simulink model "battery_simulink_model"  (R2021b)
settings: Solver=VariableStepAuto  StartTime=0.0  StopTime=14400  RelTol=1e-3
undefined symbols (not defined in the file or in its folder): Ion, Lithium
libraries: spsBatteryLib x10, spsIdealSwitchLib x4, spsCurrentMeasurementLib x3, spsParallelRLCBranchLib x2, spsControlledCurrentSourceLib x1, spspowerguiLib x1
settings Model: Creator=11  LastModifiedBy=11

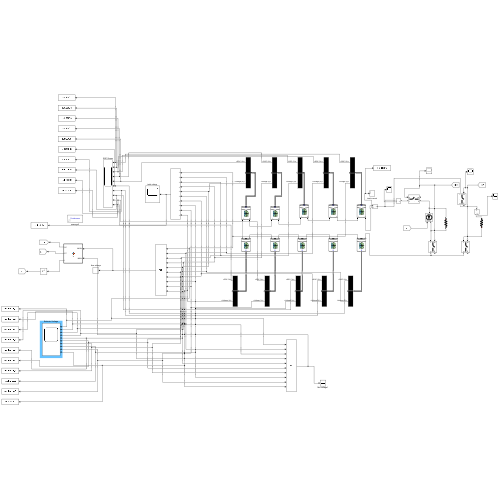
[thumbnail: Simulink's stored preview of the top-level diagram]
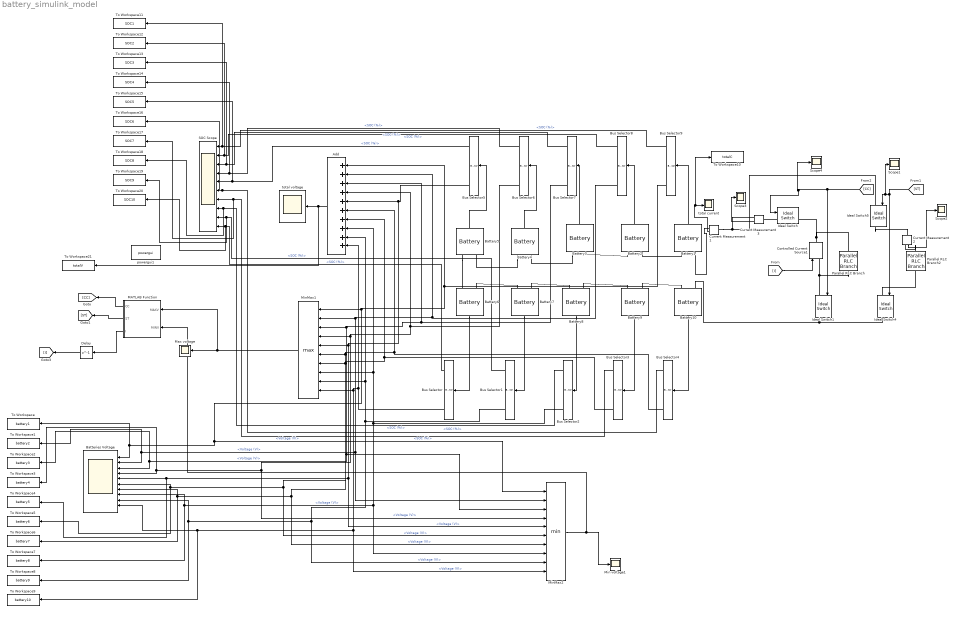
== system battery_simulink_model ==
  Add : Sum  Inputs=++++++++++
  Batteries Voltage : Scope  NumInputPorts=10
  Battery1 : spsBatteryLib/Battery  BatType=Lithium-Ion  ShowTempParam=off  ThermalPreset=no  ShowAgeParam=off  NomV=3.2  NomQ=226.1  SOC=5  Batt_Tr=30  PresetModel=off  MaxQ=226.1  MinV=2.5  FullV=3.65  Dis_rate=114  R=0.0002289  Normal_OP=203.49  expZone=[3.45,10]  current=[114]  Units=Time  Tci=20  NomT=20  T2=-30  MaxQ2=4.8  FullV2=7.1  Normal_OP2=5.655  expZone2="[6.58           1]"  Rca=0.6  ti=2000  Dp=0  Neq0=0  Tsim=1e6  Ta1=25  Qeol=5.4*0.9  Reol=0.013333*1.2  Char_age=[2.3478, 3]  Dis_age=[2.3478, 10]  N1=1500  N2=10500  N3=1000  N4=1400  Ta2=45  N5=950
  Battery10 : spsBatteryLib/Battery  BatType=Lithium-Ion  ShowTempParam=off  ThermalPreset=no  ShowAgeParam=off  NomV=3.2  NomQ=233.3  SOC=11  Batt_Tr=30  PresetModel=off  MaxQ=233.3  MinV=2.5  FullV=3.65  Dis_rate=114  R=0.0002189  Normal_OP=209.97  expZone=[3.45,10]  current=[114]  Units=Time  Tci=20  NomT=20  T2=-30  MaxQ2=4.8  FullV2=7.1  Normal_OP2=5.655  expZone2="[6.58           1]"  Rca=0.6  ti=2000  Dp=0  Neq0=0  Tsim=1e6  Ta1=25  Qeol=5.4*0.9  Reol=0.013333*1.2  Char_age=[2.3478, 3]  Dis_age=[2.3478, 10]  N1=1500  N2=10500  N3=1000  N4=1400  Ta2=45  N5=950
  Battery2 : spsBatteryLib/Battery  BatType=Lithium-Ion  ShowTempParam=off  ThermalPreset=no  ShowAgeParam=off  NomV=3.2  NomQ=238.1  SOC=10  Batt_Tr=30  PresetModel=off  MaxQ=238.1  MinV=2.5  FullV=3.65  Dis_rate=114  R=0.0002198  Normal_OP=214.29  expZone=[3.45,10]  current=[114]  Units=Time  Tci=20  NomT=20  T2=-30  MaxQ2=4.8  FullV2=7.1  Normal_OP2=5.655  expZone2="[6.58           1]"  Rca=0.6  ti=2000  Dp=0  Neq0=0  Tsim=1e6  Ta1=25  Qeol=5.4*0.9  Reol=0.013333*1.2  Char_age=[2.3478, 3]  Dis_age=[2.3478, 10]  N1=1500  N2=10500  N3=1000  N4=1400  Ta2=45  N5=950
  Battery3 : spsBatteryLib/Battery  BatType=Lithium-Ion  ShowTempParam=off  ThermalPreset=no  ShowAgeParam=off  NomV=3.2  NomQ=224.3  SOC=14  Batt_Tr=30  PresetModel=off  MaxQ=224.3  MinV=2.5  FullV=3.65  Dis_rate=114  R=0.0002171  Normal_OP=201.87  expZone=[3.45,10]  current=[114]  Units=Time  Tci=20  NomT=20  T2=-30  MaxQ2=4.8  FullV2=7.1  Normal_OP2=5.655  expZone2="[6.58           1]"  Rca=0.6  ti=2000  Dp=0  Neq0=0  Tsim=1e6  Ta1=25  Qeol=5.4*0.9  Reol=0.013333*1.2  Char_age=[2.3478, 3]  Dis_age=[2.3478, 10]  N1=1500  N2=10500  N3=1000  N4=1400  Ta2=45  N5=950
  Battery4 : spsBatteryLib/Battery  BatType=Lithium-Ion  ShowTempParam=off  ThermalPreset=no  ShowAgeParam=off  NomV=3.2  NomQ=219.1  SOC=13  Batt_Tr=30  PresetModel=off  MaxQ=219.1  MinV=2.5  FullV=3.65  Dis_rate=114  R=0.0002176  Normal_OP=197.19  expZone=[3.45,10]  current=[114]  Units=Time  Tci=20  NomT=20  T2=-30  MaxQ2=4.8  FullV2=7.1  Normal_OP2=5.655  expZone2="[6.58           1]"  Rca=0.6  ti=2000  Dp=0  Neq0=0  Tsim=1e6  Ta1=25  Qeol=5.4*0.9  Reol=0.013333*1.2  Char_age=[2.3478, 3]  Dis_age=[2.3478, 10]  N1=1500  N2=10500  N3=1000  N4=1400  Ta2=45  N5=950
  Battery5 : spsBatteryLib/Battery  BatType=Lithium-Ion  ShowTempParam=off  ThermalPreset=no  ShowAgeParam=off  NomV=3.2  NomQ=222.1  SOC=9  Batt_Tr=30  PresetModel=off  MaxQ=222.1  MinV=2.5  FullV=3.65  Dis_rate=114  R=0.0002111  Normal_OP=199.89  expZone=[3.45,10]  current=[114]  Units=Time  Tci=20  NomT=20  T2=-30  MaxQ2=4.8  FullV2=7.1  Normal_OP2=5.655  expZone2="[6.58           1]"  Rca=0.6  ti=2000  Dp=0  Neq0=0  Tsim=1e6  Ta1=25  Qeol=5.4*0.9  Reol=0.013333*1.2  Char_age=[2.3478, 3]  Dis_age=[2.3478, 10]  N1=1500  N2=10500  N3=1000  N4=1400  Ta2=45  N5=950
  Battery6 : spsBatteryLib/Battery  BatType=Lithium-Ion  ShowTempParam=off  ThermalPreset=no  ShowAgeParam=off  NomV=3.2  NomQ=219.6  SOC=14  Batt_Tr=30  PresetModel=off  MaxQ=219.6  MinV=2.5  FullV=3.65  Dis_rate=114  R=0.00023  Normal_OP=197.64  expZone=[3.45,10]  current=[114]  Units=Time  Tci=20  NomT=20  T2=-30  MaxQ2=4.8  FullV2=7.1  Normal_OP2=5.655  expZone2="[6.58           1]"  Rca=0.6  ti=2000  Dp=0  Neq0=0  Tsim=1e6  Ta1=25  Qeol=5.4*0.9  Reol=0.013333*1.2  Char_age=[2.3478, 3]  Dis_age=[2.3478, 10]  N1=1500  N2=10500  N3=1000  N4=1400  Ta2=45  N5=950
  Battery7 : spsBatteryLib/Battery  BatType=Lithium-Ion  ShowTempParam=off  ThermalPreset=no  ShowAgeParam=off  NomV=3.2  NomQ=229.7  SOC=6  Batt_Tr=30  PresetModel=off  MaxQ=229.7  MinV=2.5  FullV=3.65  Dis_rate=114  R=0.0002142  Normal_OP=206.73  expZone=[3.45,10]  current=[114]  Units=Time  Tci=20  NomT=20  T2=-30  MaxQ2=4.8  FullV2=7.1  Normal_OP2=5.655  expZone2="[6.58           1]"  Rca=0.6  ti=2000  Dp=0  Neq0=0  Tsim=1e6  Ta1=25  Qeol=5.4*0.9  Reol=0.013333*1.2  Char_age=[2.3478, 3]  Dis_age=[2.3478, 10]  N1=1500  N2=10500  N3=1000  N4=1400  Ta2=45  N5=950
  Battery8 : spsBatteryLib/Battery  BatType=Lithium-Ion  ShowTempParam=off  ThermalPreset=no  ShowAgeParam=off  NomV=3.2  NomQ=224.7  SOC=13  Batt_Tr=30  PresetModel=off  MaxQ=224.7  MinV=2.5  FullV=3.65  Dis_rate=114  R=0.0002093  Normal_OP=202.23  expZone=[3.45,10]  current=[114]  Units=Time  Tci=20  NomT=20  T2=-30  MaxQ2=4.8  FullV2=7.1  Normal_OP2=5.655  expZone2="[6.58           1]"  Rca=0.6  ti=2000  Dp=0  Neq0=0  Tsim=1e6  Ta1=25  Qeol=5.4*0.9  Reol=0.013333*1.2  Char_age=[2.3478, 3]  Dis_age=[2.3478, 10]  N1=1500  N2=10500  N3=1000  N4=1400  Ta2=45  N5=950
  Battery9 : spsBatteryLib/Battery  BatType=Lithium-Ion  ShowTempParam=off  ThermalPreset=no  ShowAgeParam=off  NomV=3.2  NomQ=217.6  SOC=7  Batt_Tr=30  PresetModel=off  MaxQ=217.6  MinV=2.5  FullV=3.65  Dis_rate=114  R=0.0002233  Normal_OP=195.84  expZone=[3.45,10]  current=[114]  Units=Time  Tci=20  NomT=20  T2=-30  MaxQ2=4.8  FullV2=7.1  Normal_OP2=5.655  expZone2="[6.58           1]"  Rca=0.6  ti=2000  Dp=0  Neq0=0  Tsim=1e6  Ta1=25  Qeol=5.4*0.9  Reol=0.013333*1.2  Char_age=[2.3478, 3]  Dis_age=[2.3478, 10]  N1=1500  N2=10500  N3=1000  N4=1400  Ta2=45  N5=950
  Bus Selector{,1..9} (10 alike) : BusSelector  OutputSignals=SOC (%),Current (A),Voltage (V)
  Controlled Current Source1 : spsControlledCurrentSourceLib/Controlled Current Source  Initialize=on  Source_Type=DC  Amplitude=0  Phase=0  Frequency=0  Measurements=None
  Current Measurement1 : spsCurrentMeasurementLib/Current Measurement  PhasorSimulation=off  OutputType=Complex  PSBequivalent=0
  Current Measurement2 : spsCurrentMeasurementLib/Current Measurement  PhasorSimulation=off  OutputType=Complex  PSBequivalent=0
  Current Measurement3 : spsCurrentMeasurementLib/Current Measurement  PhasorSimulation=off  OutputType=Complex  PSBequivalent=0
  Delay : Delay  DelayLength=1  InitialCondition=0
  Ideal Switch{,1,4..5} (4 alike) : spsIdealSwitchLib/Ideal Switch  Ron=0  Lon=0  IC=0  Rs=0  Cs=0  Measurements=on
  MATLAB Function : MATLAB Function  TreatAsAtomicUnit=on  SystemSampleTime=1
  Max voltage : Scope
  Min voltage1 : Scope
  MinMax1 : MinMax  Function=max  Inputs=10
  MinMax2 : MinMax  Inputs=10
  Parallel RLC Branch : spsParallelRLCBranchLib/Parallel RLC Branch  LConnTagsString=a  RConnTagsString=__new0  BranchType=R  Resistance=1000000000  Inductance=1e-3  SetiL0=off  InitialCurrent=0  Capacitance=1e-6  Setx0=off  InitialVoltage=0  Measurements=None
  Parallel RLC Branch2 : spsParallelRLCBranchLib/Parallel RLC Branch  LConnTagsString=a  RConnTagsString=__new0  BranchType=R  Resistance=10000  Inductance=1e-3  SetiL0=off  InitialCurrent=0  Capacitance=1e-6  Setx0=off  InitialVoltage=0  Measurements=None
  SOC Scope : Scope  NumInputPorts=10
  Scope{1..4} (4 alike) : Scope
  To Workspace : ToWorkspace  VariableName=battery1  SaveFormat=Timeseries  SampleTime=-1
  To Workspace1 : ToWorkspace  VariableName=battery2  SaveFormat=Timeseries  SampleTime=-1
  To Workspace10 : ToWorkspace  VariableName=totalC  SaveFormat=Timeseries  SampleTime=-1
  To Workspace11 : ToWorkspace  VariableName=SOC1  SaveFormat=Timeseries  SampleTime=-1
  To Workspace12 : ToWorkspace  VariableName=SOC2  SaveFormat=Timeseries  SampleTime=-1
  To Workspace13 : ToWorkspace  VariableName=SOC3  SaveFormat=Timeseries  SampleTime=-1
  To Workspace14 : ToWorkspace  VariableName=SOC4  SaveFormat=Timeseries  SampleTime=-1
  To Workspace15 : ToWorkspace  VariableName=SOC5  SaveFormat=Timeseries  SampleTime=-1
  To Workspace16 : ToWorkspace  VariableName=SOC6  SaveFormat=Timeseries  SampleTime=-1
  To Workspace17 : ToWorkspace  VariableName=SOC7  SaveFormat=Timeseries  SampleTime=-1
  To Workspace18 : ToWorkspace  VariableName=SOC8  SaveFormat=Timeseries  SampleTime=-1
  To Workspace19 : ToWorkspace  VariableName=SOC9  SaveFormat=Timeseries  SampleTime=-1
  To Workspace2 : ToWorkspace  VariableName=battery3  SaveFormat=Timeseries  SampleTime=-1
  To Workspace20 : ToWorkspace  VariableName=SOC10  SaveFormat=Timeseries  SampleTime=-1
  To Workspace21 : ToWorkspace  VariableName=totalV  SaveFormat=Timeseries  SampleTime=-1
  To Workspace3 : ToWorkspace  VariableName=battery4  SaveFormat=Timeseries  SampleTime=-1
  To Workspace4 : ToWorkspace  VariableName=battery5  SaveFormat=Timeseries  SampleTime=-1
  To Workspace5 : ToWorkspace  VariableName=battery6  SaveFormat=Timeseries  SampleTime=-1
  To Workspace6 : ToWorkspace  VariableName=battery7  SaveFormat=Timeseries  SampleTime=-1
  To Workspace7 : ToWorkspace  VariableName=battery8  SaveFormat=Timeseries  SampleTime=-1
  To Workspace8 : ToWorkspace  VariableName=battery9  SaveFormat=Timeseries  SampleTime=-1
  To Workspace9 : ToWorkspace  VariableName=battery10  SaveFormat=Timeseries  SampleTime=-1
  powergui1 : spspowerguiLib/powergui  Priority=1  SimulationMode=Continuous  SampleTime=50e-6  frequency=60  Iterations=50  frequencyindice=0  Pbase=100e6  ErrMax=1e-4  UnitsV=kV  UnitsW=MW  buscounter=0  FunctionMessages=off  echomessages=off  EnableUseOfTLC=off  CurrentSourceSwitches=off  DisableSnubberDevices=off  DisableRonSwitches=off  DisableVfSwitches=off  DisplayEquations=off  AutomaticDiscreteSolvers=off  SolverType=Tustin/Backward Euler (TBE)  Interpol=off  ExternalGateDelay=off  methode=off  Ts=100  x0status=blocks  SPID=on  SwTol=0  HookPort=off  NonlinearTolerance=1e-4  nMaxIteration=100  ContinueOnMaxIteration=off  RestoreLinks=warning  ResistiveCurrentMeasurement=off  Frange=[0:2:500]  Ylog=off  Xlog=on  ShowGrid=off  save=off  variable=ZData  structure=0  ZoomFFT=off  StartTime=0.0  cycles=1  DisplayStyle=1  fundamental=60  FreqAxis=off  MaxFrequency=1000  frequencyindicesteady=1  RmsSteady=1  display=off
  total current : Scope
  total voltage : Scope
  wires:
  Bus Selector9/1 -> To Workspace11/1, SOC Scope/1  "<SOC (%)>"
  Battery4/1 -> Bus Selector6/1
  Battery9/1 -> Bus Selector3/1
  Delay/1 -> [I]
  Bus Selector1/3 -> MinMax2/9, To Workspace8/1, Batteries Voltage/9, Add/9, MinMax1/9  "<Voltage (V)>"
  MATLAB Function/3(I) -> Delay/1
  Battery7/1 -> Bus Selector1/1
  [I] -> Controlled Current Source1/1
  Current Measurement1/1 -> To Workspace10/1, total current/1
  Battery10/1 -> Bus Selector4/1
  Current Measurement2/1 -> Scope2/1
  MATLAB Function/2(ST) -> [ST]
  Bus Selector/3 -> Add/10, To Workspace9/1, Batteries Voltage/10, MinMax2/10, MinMax1/10  "<Voltage (V)>"
  [CC] -> Ideal Switch1/1, Ideal Switch/1, Scope4/1
  MATLAB Function/1(CC) -> [CC]
  Bus Selector3/1 -> To Workspace17/1, SOC Scope/7  "<SOC (%)>"
  Bus Selector3/3 -> MinMax2/7, To Workspace6/1, Batteries Voltage/7, MinMax1/7, Add/7  "<Voltage (V)>"
  Bus Selector2/1 -> To Workspace18/1, SOC Scope/8  "<SOC (%)>"
  Bus Selector9/3 -> Add/1, MinMax2/1, To Workspace/1, Batteries Voltage/1, MinMax1/1  "<Voltage (V)>"
  [ST] -> Ideal Switch4/1, Scope1/1, Ideal Switch5/1
  Bus Selector5/1 -> To Workspace15/1, SOC Scope/5  "<SOC (%)>"
  Battery5/1 -> Bus Selector5/1
  Battery3/1 -> Bus Selector7/1
  Bus Selector4/1 -> To Workspace16/1, SOC Scope/6  "<SOC (%)>"
  Battery6/1 -> Bus Selector/1
  Current Measurement3/1 -> Scope3/1
  MinMax2/1 -> MATLAB Function/2(MINV), Min voltage1/1
  Bus Selector/1 -> To Workspace20/1, SOC Scope/10  "<SOC (%)>"
  Bus Selector6/1 -> To Workspace14/1, SOC Scope/4  "<SOC (%)>"
  Bus Selector4/3 -> Add/6, MinMax2/6, To Workspace5/1, Batteries Voltage/6, MinMax1/6  "<Voltage (V)>"
  Bus Selector2/3 -> MinMax2/8, To Workspace7/1, Batteries Voltage/8, Add/8, MinMax1/8  "<Voltage (V)>"
  Add/1 -> To Workspace21/1, total voltage/1
  Bus Selector7/3 -> To Workspace2/1, Batteries Voltage/3, MinMax2/3, MinMax1/3, Add/3  "<Voltage (V)>"
  Bus Selector1/1 -> To Workspace19/1, SOC Scope/9  "<SOC (%)>"
  Bus Selector7/1 -> SOC Scope/3, To Workspace13/1  "<SOC (%)>"
  Battery2/1 -> Bus Selector8/1
  MinMax1/1 -> Max voltage/1, MATLAB Function/1(MAXV)
  Bus Selector8/3 -> Add/2, MinMax2/2, To Workspace1/1, Batteries Voltage/2, MinMax1/2  "<Voltage (V)>"
  Battery8/1 -> Bus Selector2/1
  Bus Selector8/1 -> To Workspace12/1, SOC Scope/2  "<SOC (%)>"
  Bus Selector5/3 -> MinMax2/5, To Workspace4/1, Batteries Voltage/5, MinMax1/5, Add/5  "<Voltage (V)>"
  Bus Selector6/3 -> Add/4, MinMax2/4, To Workspace3/1, Batteries Voltage/4, MinMax1/4  "<Voltage (V)>"
  Battery1/1 -> Bus Selector9/1
  connections:
  Ideal Switch5/LConn1 -- Current Measurement1/LConn1 -- Current Measurement3/RConn1
  Controlled Current Source1/RConn1 -- Parallel RLC Branch/LConn1 -- Ideal Switch/RConn1
  Ideal Switch1/LConn1 -- Parallel RLC Branch/RConn1 -- Controlled Current Source1/LConn1
  Ideal Switch1/RConn1 -- Ideal Switch4/RConn1 -- Battery10/LConn2
  Battery1/LConn2 -- Battery2/LConn1
  Battery3/LConn2 -- Battery4/LConn1
  Battery5/LConn2 -- Battery6/LConn1
  Current Measurement1/RConn1 -- Battery1/LConn1
  Battery8/LConn2 -- Battery9/LConn1
  Battery4/LConn2 -- Battery5/LConn1
  Ideal Switch5/RConn1 -- Current Measurement2/LConn1
  Battery7/LConn2 -- Battery8/LConn1
  Battery6/LConn2 -- Battery7/LConn1
  Parallel RLC Branch2/RConn1 -- Current Measurement2/RConn1
  Battery2/LConn2 -- Battery3/LConn1
  Ideal Switch/LConn1 -- Current Measurement3/LConn1
  Ideal Switch4/LConn1 -- Parallel RLC Branch2/LConn1
  Battery9/LConn2 -- Battery10/LConn1

== matlab function battery_simulink_model/MATLAB Function ==
  data: MAXV input; MINV input; CC output; ST output; I output
function [CC, ST,I]  = fcn(MAXV,MINV)
persistent state charge_state count;

CC = 0;
ST = 0;
I = 0;
%初始化
if isempty(state)
    state = 2;
    I = 0;
    charge_state = 1;
    count = 0;
end

%充放电循环
if MAXV >= 3.65
    charge_state = 0;
    count = 300;
elseif MINV <= 2.85
    charge_state = 1;
    count = 300;
end

if charge_state == 1%充电循环
    if count == 0
        I = 0.5*228;
        state = 1;
    else
        count = count -1;
        state = 2
    end

elseif charge_state == 0%放电循环
    if count == 0
        I = -0.5*228;
        state = 1;
    else
        count = count -1;
        state = 2;
    end
end

switch state
    case 1
        CC = 1;
        ST = 0;
    case 2
        CC = 0;
        ST = 1;
    case 3
        CC = 0;
        ST = 0;
end
